simulink model "Testing_model"  (R2024b)
settings: Solver=FixedStepAuto  StartTime=0.0  StopTime=2  FixedStep=50e-6  RelTol=1e-3
undefined symbols (not defined in the file): alpha_Lpf, B, dspblkCoreblockFVToolHelper, gcbh, J, Ki_current, Ki_speed, Kp_current, Kp_speed, lamdaM, Ls, ma, P, Rs, T_max, Ts, Vdc
libraries: simulink x3, slpidlib x3, eeGeneralControl x1
settings Model: Creator=ahmed  LastModifiedBy=ahmed

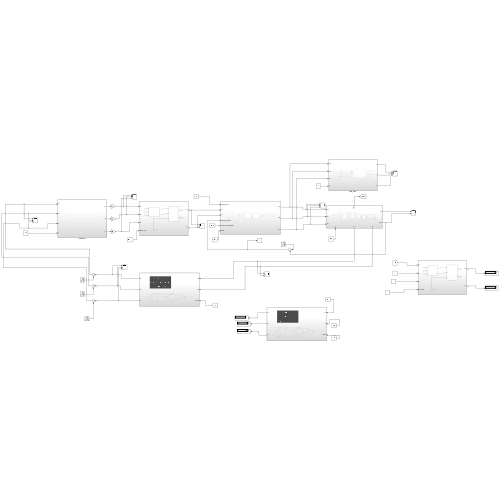
[thumbnail: Simulink's stored preview of the top-level diagram]
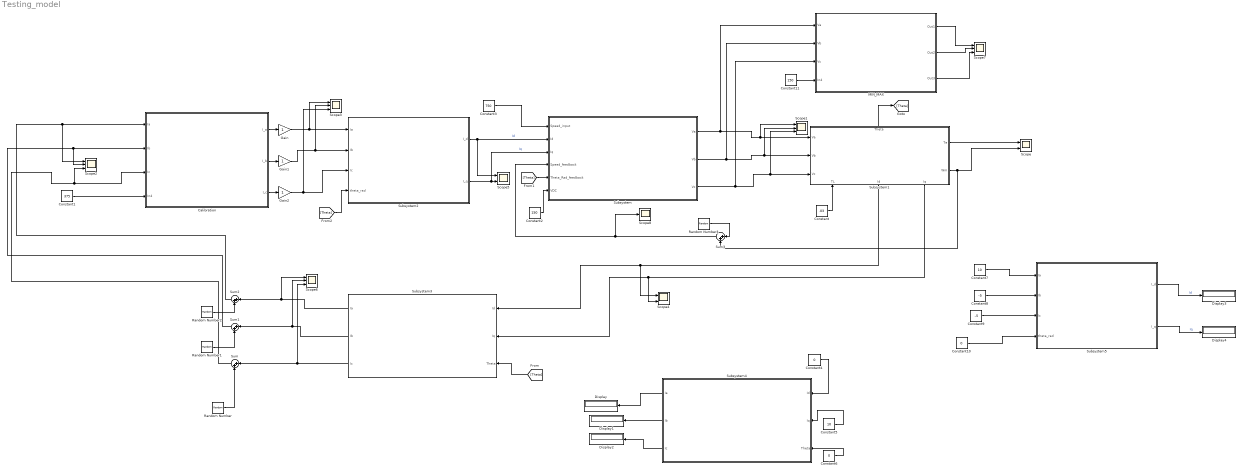
== system Testing_model ==
  Calibration : Subsystem
  Constant : Constant  Value=.03
  Constant1 : Constant  Value=375
  Constant10 : Constant  Value=0
  Constant11 : Constant  Value=150
  Constant2 : Constant  Value=150
  Constant3 : Constant  Value=750
  Constant4 : Constant  Value=0
  Constant5 : Constant  Value=10
  Constant6 : Constant  Value=0
  Constant7 : Constant  Value=10
  Constant8 : Constant  Value=-5
  Constant9 : Constant  Value=-5
  Display{,1..4} (5 alike) : Display
  Gain : Gain
  Gain1 : Gain
  Gain2 : Gain
  MIN_MAX : Subsystem
  Random Number : RandomNumber  Variance=.005  SampleTime=Ts
  Random Number1 : RandomNumber  Variance=.005  SampleTime=Ts
  Random Number2 : RandomNumber  Variance=.005  SampleTime=Ts
  Random Number3 : RandomNumber  Variance=50  SampleTime=Ts
  Scope : Scope  NumInputPorts=2
  Scope{1..3,6..7} (5 alike) : Scope  NumInputPorts=3
  Scope4 : Scope  NumInputPorts=2
  Scope5 : Scope  NumInputPorts=2
  Scope8 : Scope
  Subsystem : Subsystem
  Subsystem1 : Subsystem
      settings: PortSchema="{\"entries\":[{\"content\":{\"sides\":[{\"content\":{\"connectorIds\":[\"In1\",\"In2\",\"In3\"]},\"type\":\"ConnectorPlacement.EquallySpacedRectSide\",\"uuid\":\"410fafe1-6d3d-4b62-9ccb-454f6008b81a\"},{\"content\":{\"connectorIds\":[\"Out1\",\"Out2\"],\"side\":\"RIGHT\"},\"type\":\"ConnectorPlacement.EquallySpacedRectSide\",\"uuid\":\"b4215a85-6f2a-4bbd-a305-1fa3c25faaac\"},{\"content\":{\"connectorIds\":[\"Out5\"],\"side\":\"TOP\"},\"type\":\"ConnectorPlacement.EquallySpacedRectSide\",\"uuid\":\"c3471a58-e27d-4fa8-ab5e-4301d929309b\"},{\"content\":{\"connectorIds\":[\"In4\",\"Out3\",\"Out4\"],\"side\":\"BOTTOM\"},\"type\":\"ConnectorPlacement.EquallySpacedRectSide\",\"uuid\":\"92e7eecc-1ce6-457d-b998-008a2505e29d\"}]},\"type\":\"ConnectorPlacement.EquallySpacedConnector\",\"uuid\":\"8b1e994c-6614-4fb4-bf28-22b9fb88c59f\"}],\"packageUris\":[\"http://schema.mathworks.com/mf0/Connector/R2020b\"],\"version\":\"1.0\"}"
  Subsystem2 : Subsystem
  Subsystem3 : Subsystem
  Subsystem4 : Subsystem
  Subsystem5 : Subsystem
  Sum{,1..3} (4 alike) : Sum  Inputs=|++
  wires:
  Subsystem/1(Va) -> MIN_MAX/1(Va), Scope1/1, Subsystem1/1(Va)
  Subsystem/2(Vb) -> MIN_MAX/2(Vb), Scope1/2, Subsystem1/2(Vb)
  Subsystem/3(Vc) -> MIN_MAX/3(Vc), Scope1/3, Subsystem1/3(Vc)
  Subsystem1/5(Theta) -> [Theta]
  Constant/1 -> Subsystem1/4(TL)
  Subsystem1/1(Te) -> Scope/1
  Subsystem1/2(Wm) -> Scope/2, Sum3/2
  [Theta] -> Subsystem3/3(Theta)
  Constant1/1 -> Calibration/4(In4)
  [Theta] -> Subsystem/5(Theta_Rad_feedback)
  Constant2/1 -> Subsystem/6(VDC)
  Constant3/1 -> Subsystem/1(Speed_input)
  Random Number/1 -> Sum/2
  Subsystem3/3(Ic) -> Scope6/3, Sum/1
  Subsystem3/2(Ib) -> Sum1/1, Scope6/2
  Random Number1/1 -> Sum1/2
  Subsystem3/1(Ia) -> Scope6/1, Sum2/1
  Random Number2/1 -> Sum2/2
  [Theta] -> Subsystem2/4(theta_rad)
  Subsystem1/3(Id) -> Scope4/1, Subsystem3/1(Id)
  Subsystem1/4(Iq) -> Scope4/2, Subsystem3/2(Iq)
  Sum2/1 -> Scope2/1, Calibration/1(Ia)
  Sum1/1 -> Scope2/2, Calibration/2(Ib)
  Sum/1 -> Scope2/3, Calibration/3(Ic)
  Subsystem2/1(I_d) -> Scope5/1, Subsystem/2(Id)  "Id"
  Subsystem2/2(I_q) -> Scope5/2, Subsystem/3(Iq)  "Iq"
  Constant4/1 -> Subsystem4/1(Id)
  Constant5/1 -> Subsystem4/2(Iq)
  Constant6/1 -> Subsystem4/3(Theta)
  Subsystem4/1(Ia) -> Display/1
  Subsystem4/2(Ib) -> Display1/1
  Subsystem4/3(Ic) -> Display2/1
  Constant7/1 -> Subsystem5/1(Ia)
  Constant9/1 -> Subsystem5/3(Ic)
  Constant8/1 -> Subsystem5/2(Ib)
  Constant10/1 -> Subsystem5/4(theta_rad)
  Subsystem5/1(I_d) -> Display3/1  "Id"
  Subsystem5/2(I_q) -> Display4/1  "Iq"
  Calibration/2(I_b) -> Gain1/1
  Calibration/1(I_a) -> Gain/1
  Calibration/3(I_c) -> Gain2/1
  Gain/1 -> Subsystem2/1(Ia), Scope3/1
  Gain1/1 -> Scope3/2, Subsystem2/2(Ib)
  Gain2/1 -> Subsystem2/3(Ic), Scope3/3
  Constant11/1 -> MIN_MAX/4(In4)
  MIN_MAX/1(Out1) -> Scope7/1
  MIN_MAX/2(Out2) -> Scope7/2
  MIN_MAX/3(Out3) -> Scope7/3
  Sum3/1 -> Scope8/1, Subsystem/4(Speed_feedback)
  Random Number3/1 -> Sum3/1

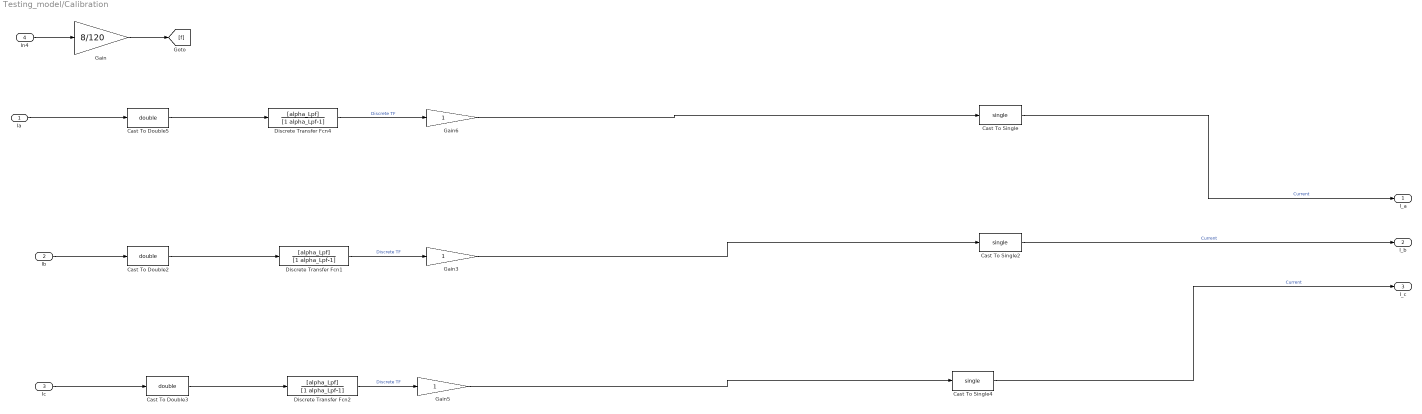
== system Testing_model/Calibration ==
  Ia : Inport
  Ib : Inport  Port=2
  Ic : Inport  Port=3
  In4 : Inport  Port=4
  Cast To Double2 : DataTypeConversion  OutDataTypeStr=double  SaturateOnIntegerOverflow=off  RndMeth=Floor
  Cast To Double3 : DataTypeConversion  OutDataTypeStr=double  SaturateOnIntegerOverflow=off  RndMeth=Floor
  Cast To Double5 : DataTypeConversion  OutDataTypeStr=double  SaturateOnIntegerOverflow=off  RndMeth=Floor
  Cast To Single : DataTypeConversion  OutDataTypeStr=single  SaturateOnIntegerOverflow=off  RndMeth=Floor
  Cast To Single2 : DataTypeConversion  OutDataTypeStr=single  SaturateOnIntegerOverflow=off  RndMeth=Floor
  Cast To Single4 : DataTypeConversion  OutDataTypeStr=single  SaturateOnIntegerOverflow=off  RndMeth=Floor
  Discrete Transfer Fcn1 : DiscreteTransferFcn  LoadFcn=dspblkCoreblockFVToolHelper(gcbh,'load');  Numerator=[alpha_Lpf]  Denominator=[1 alpha_Lpf-1]  RndMeth=Nearest
      settings: CopyFcn=dspblkCoreblockFVToolHelper(gcbh,'copy');  DeleteFcn=dspblkCoreblockFVToolHelper(gcbh,'close');  ModelCloseFcn=dspblkCoreblockFVToolHelper(gcbh,'close');  PreSaveFcn=dspblkCoreblockFVToolHelper(gcbh,'presave');  PostSaveFcn=dspblkCoreblockFVToolHelper(gcbh,'postsave');  CloseFcn=dspblkCoreblockFVToolHelper(gcbh,'close');
  Discrete Transfer Fcn2 : DiscreteTransferFcn  LoadFcn=dspblkCoreblockFVToolHelper(gcbh,'load');  Numerator=[alpha_Lpf]  Denominator=[1 alpha_Lpf-1]  RndMeth=Nearest
      settings: CopyFcn=dspblkCoreblockFVToolHelper(gcbh,'copy');  DeleteFcn=dspblkCoreblockFVToolHelper(gcbh,'close');  ModelCloseFcn=dspblkCoreblockFVToolHelper(gcbh,'close');  PreSaveFcn=dspblkCoreblockFVToolHelper(gcbh,'presave');  PostSaveFcn=dspblkCoreblockFVToolHelper(gcbh,'postsave');  CloseFcn=dspblkCoreblockFVToolHelper(gcbh,'close');
  Discrete Transfer Fcn4 : DiscreteTransferFcn  LoadFcn=dspblkCoreblockFVToolHelper(gcbh,'load');  Numerator=[alpha_Lpf]  Denominator=[1 alpha_Lpf-1]  RndMeth=Nearest
      settings: CopyFcn=dspblkCoreblockFVToolHelper(gcbh,'copy');  DeleteFcn=dspblkCoreblockFVToolHelper(gcbh,'close');  ModelCloseFcn=dspblkCoreblockFVToolHelper(gcbh,'close');  PreSaveFcn=dspblkCoreblockFVToolHelper(gcbh,'presave');  PostSaveFcn=dspblkCoreblockFVToolHelper(gcbh,'postsave');  CloseFcn=dspblkCoreblockFVToolHelper(gcbh,'close');
  Gain : Gain  Gain=8/120
  Gain3 : Gain
  Gain5 : Gain
  Gain6 : Gain
  I_a : Outport
  I_b : Outport  Port=2
  I_c : Outport  Port=3
  wires:
  Ib/1 -> Cast To Double2/1
  Gain3/1 -> Cast To Single2/1
  Discrete Transfer Fcn1/1 -> Gain3/1  "Discrete TF"
  Gain6/1 -> Cast To Single/1
  Gain5/1 -> Cast To Single4/1
  Cast To Double2/1 -> Discrete Transfer Fcn1/1
  Discrete Transfer Fcn4/1 -> Gain6/1  "Discrete TF"
  Cast To Double5/1 -> Discrete Transfer Fcn4/1
  Discrete Transfer Fcn2/1 -> Gain5/1  "Discrete TF"
  Cast To Single2/1 -> I_b/1  "Current"
  Cast To Double3/1 -> Discrete Transfer Fcn2/1
  Ia/1 -> Cast To Double5/1
  Cast To Single/1 -> I_a/1  "Current"
  Cast To Single4/1 -> I_c/1  "Current"
  Ic/1 -> Cast To Double3/1
  In4/1 -> Gain/1
  Gain/1 -> [f]

== system Testing_model/MIN_MAX ==
  Va : Inport
  Vb : Inport  Port=2
  Vc : Inport  Port=3
  In4 : Inport  Port=4
  Divide : Product  Inputs=*/
  Divide1 : Product  Inputs=*/
  Divide2 : Product  Inputs=*/
  Gain : Gain  Gain=1/sqrt(3)
  MIN_MAX : Subsystem
  Saturation : Saturate  UpperLimit=95  LowerLimit=0
  Saturation1 : Saturate  UpperLimit=95  LowerLimit=0
  Saturation2 : Saturate  UpperLimit=95  LowerLimit=0
  Scope2 : Scope  NumInputPorts=3
  Out1 : Outport
  Out2 : Outport  Port=2
  Out3 : Outport  Port=3
  wires:
  Saturation/1 -> Out1/1
  Saturation1/1 -> Out2/1
  Saturation2/1 -> Out3/1
  Va/1 -> Divide2/1
  Vb/1 -> Divide1/1
  Vc/1 -> Divide/1
  Divide2/1 -> MIN_MAX/1(In1), Scope2/1
  Divide1/1 -> Scope2/2, MIN_MAX/2(In2)
  Divide/1 -> Scope2/3, MIN_MAX/3(In3)
  In4/1 -> Gain/1
  Gain/1 -> Divide2/2, Divide1/2, Divide/2
  MIN_MAX/1(Out1) -> Saturation/1
  MIN_MAX/2(Out2) -> Saturation1/1
  MIN_MAX/3(Out3) -> Saturation2/1

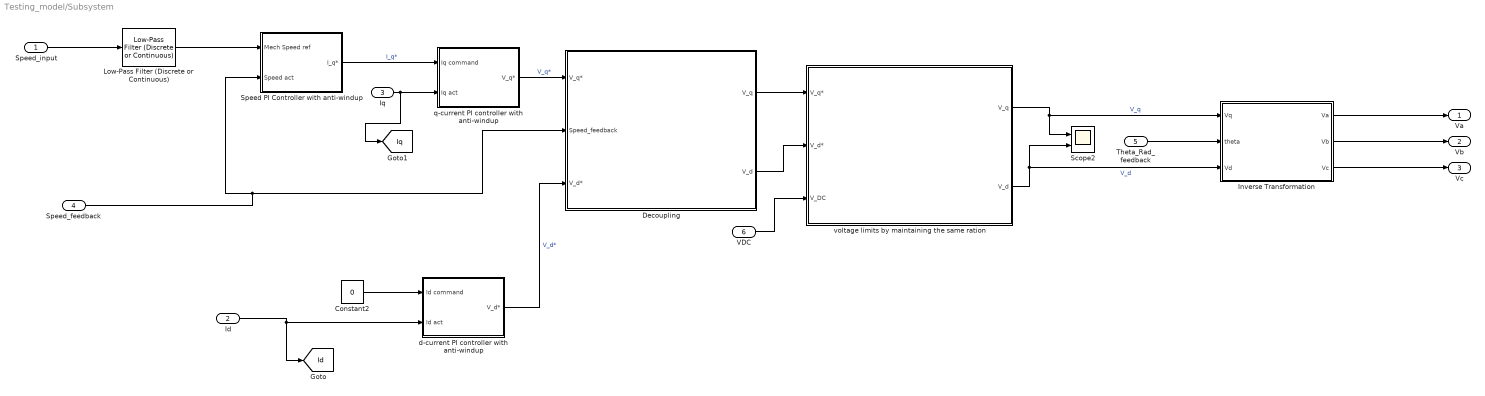
== system Testing_model/Subsystem ==
  Speed_input : Inport
  Id : Inport  Port=2
  Iq : Inport  Port=3
  Speed_feedback : Inport  Port=4
  Theta_Rad_feedback : Inport  Port=5
  VDC : Inport  Port=6
  Constant2 : Constant  Value=0  SampleTime=Ts
  Decoupling : Subsystem
  Inverse Transformation : Subsystem
  Low-Pass Filter (Discrete or Continuous) : eeGeneralControl/Low-Pass Filter (Discrete or Continuous)  K=1  T=1/60  B=inf  A=-inf  init_option=Inherited from block input  x0=0  Ts=-1
  Scope2 : Scope  NumInputPorts=2
  Speed PI Controller with anti-windup : Subsystem
  d-current PI controller with anti-windup : Subsystem
  q-current PI controller with anti-windup : Subsystem
  voltage limits by maintaining the same ration : Subsystem
  Va : Outport
  Vb : Outport  Port=2
  Vc : Outport  Port=3
  tag scope: Id=global, Iq=global
  wires:
  Speed_feedback/1 -> Decoupling/2(Speed_feedback), Speed PI Controller with anti-windup/2(Speed act)
  Speed_input/1 -> Low-Pass Filter (Discrete or Continuous)/1
  Iq/1 -> q-current PI controller with anti-windup/2(Iq act), [Iq]
  Speed PI Controller with anti-windup/1(I_q*) -> q-current PI controller with anti-windup/1(Iq command)  "I_q*"
  Constant2/1 -> d-current PI controller with anti-windup/1(Id command)
  Decoupling/2(V_d) -> voltage limits by maintaining the same ration/2(V_d*)
  Id/1 -> d-current PI controller with anti-windup/2(Id act), [Id]
  q-current PI controller with anti-windup/1(V_q*) -> Decoupling/1(V_q*)  "V_q*"
  d-current PI controller with anti-windup/1(V_d*) -> Decoupling/3(V_d*)  "V_d*"
  Decoupling/1(V_q) -> voltage limits by maintaining the same ration/1(V_q*)
  VDC/1 -> voltage limits by maintaining the same ration/3(V_DC)
  voltage limits by maintaining the same ration/1(V_q) -> Scope2/1, Inverse Transformation/1(Vq)  "V_q"
  voltage limits by maintaining the same ration/2(V_d) -> Inverse Transformation/3(Vd), Scope2/2  "V_d"
  Theta_Rad_feedback/1 -> Inverse Transformation/2(theta)
  Inverse Transformation/3(Vc) -> Vc/1
  Inverse Transformation/1(Va) -> Va/1
  Inverse Transformation/2(Vb) -> Vb/1
  Low-Pass Filter (Discrete or Continuous)/1 -> Speed PI Controller with anti-windup/1(Mech Speed ref)

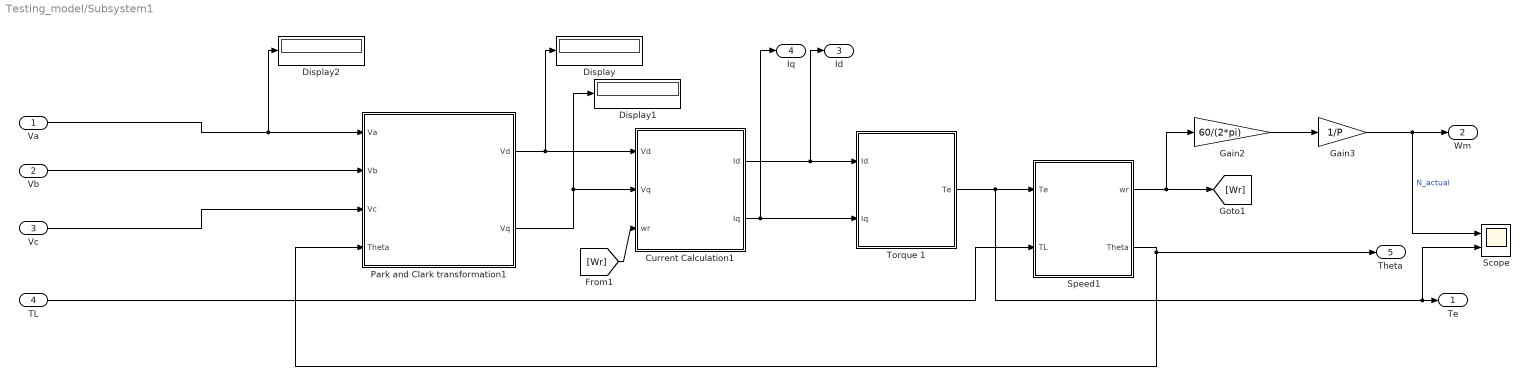
== system Testing_model/Subsystem1 ==
  Va : Inport
  Vb : Inport  Port=2
  Vc : Inport  Port=3
  TL : Inport  Port=4
  Current Calculation1 : Subsystem
  Display : Display
  Display1 : Display
  Display2 : Display
  Gain2 : Gain  Gain=60/(2*pi)
  Gain3 : Gain  Gain=1/P
  Park and Clark transformation1 : Subsystem
  Scope : Scope  NumInputPorts=2
  Speed1 : Subsystem
  Torque 1 : Subsystem
  Te : Outport
  Wm : Outport  Port=2
  Id : Outport  Port=3
  Iq : Outport  Port=4
  Theta : Outport  Port=5
  wires:
  [Wr] -> Current Calculation1/3(wr)
  Va/1 -> Display2/1, Park and Clark transformation1/1(Va)
  Park and Clark transformation1/2(Vq) -> Current Calculation1/2(Vq), Display1/1
  Torque 1/1(Te) -> Scope/2, Te/1, Speed1/1(Te)
  Speed1/1(wr) -> Gain2/1, [Wr]
  Park and Clark transformation1/1(Vd) -> Display/1, Current Calculation1/1(Vd)
  Gain2/1 -> Gain3/1
  Speed1/2(Theta) -> Park and Clark transformation1/4(Theta), Theta/1
  Current Calculation1/2(Iq) -> Torque 1/2(Iq), Iq/1
  Current Calculation1/1(Id) -> Id/1, Torque 1/1(Id)
  Vb/1 -> Park and Clark transformation1/2(Vb)
  Gain3/1 -> Scope/1, Wm/1  "N_actual"
  Vc/1 -> Park and Clark transformation1/3(Vc)
  TL/1 -> Speed1/2(TL)

== system Testing_model/Subsystem2 ==
  Ia : Inport
  Ib : Inport  Port=2
  Ic : Inport  Port=3
  theta_rad : Inport  Port=4
  Forward Clacke : Subsystem
  Forward Park : Subsystem
  I_d : Outport
  I_q : Outport  Port=2
  wires:
  Ic/1 -> Forward Clacke/3(Ic)
  Forward Clacke/2(I_beta) -> Forward Park/2(I_beta)
  Forward Clacke/1(I_alpha) -> Forward Park/1(I_alpha)
  Ia/1 -> Forward Clacke/1(Ia)
  Forward Park/1(I_d) -> I_d/1
  Forward Park/2(I_q) -> I_q/1
  Ib/1 -> Forward Clacke/2(Ib)
  theta_rad/1 -> Forward Park/3(theta_rad)

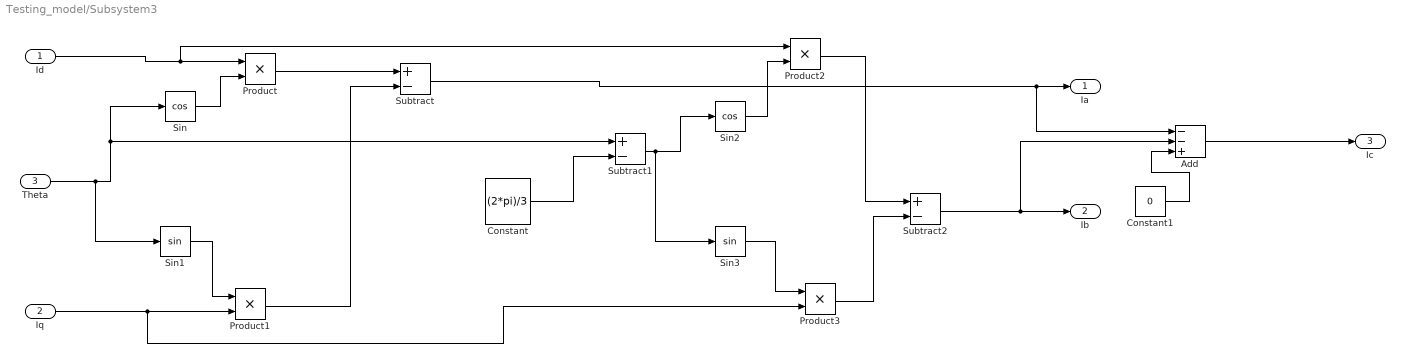
== system Testing_model/Subsystem3 ==
  Id : Inport
  Iq : Inport  Port=2
  Theta : Inport  Port=3
  Add : Sum  Inputs=--+
  Constant : Constant  Value=(2*pi)/3
  Constant1 : Constant  Value=0
  Product{,1..3} (4 alike) : Product
  Sin : Trigonometry  Operator=cos
  Sin1 : Trigonometry
  Sin2 : Trigonometry  Operator=cos
  Sin3 : Trigonometry
  Subtract : Sum  Inputs=+-
  Subtract1 : Sum  Inputs=+-
  Subtract2 : Sum  Inputs=+-
  Ia : Outport
  Ib : Outport  Port=2
  Ic : Outport  Port=3
  wires:
  Theta/1 -> Sin1/1, Sin/1, Subtract1/1
  Id/1 -> Product2/1, Product/1
  Sin/1 -> Product/2
  Product/1 -> Subtract/1
  Iq/1 -> Product3/2, Product1/2
  Sin1/1 -> Product1/1
  Product1/1 -> Subtract/2
  Subtract/1 -> Add/1, Ia/1
  Constant/1 -> Subtract1/2
  Subtract1/1 -> Sin3/1, Sin2/1
  Sin2/1 -> Product2/2
  Sin3/1 -> Product3/1
  Product3/1 -> Subtract2/2
  Product2/1 -> Subtract2/1
  Subtract2/1 -> Add/2, Ib/1
  Constant1/1 -> Add/3
  Add/1 -> Ic/1

== system Testing_model/Subsystem4 ==
  Id : Inport
  Iq : Inport  Port=2
  Theta : Inport  Port=3
  Add : Sum  Inputs=--+
  Constant : Constant  Value=(2*pi)/3
  Constant1 : Constant  Value=0
  Product{,1..3} (4 alike) : Product
  Sin : Trigonometry  Operator=cos
  Sin1 : Trigonometry
  Sin2 : Trigonometry  Operator=cos
  Sin3 : Trigonometry
  Subtract : Sum  Inputs=+-
  Subtract1 : Sum  Inputs=+-
  Subtract2 : Sum  Inputs=+-
  Ia : Outport
  Ib : Outport  Port=2
  Ic : Outport  Port=3
  wires:
  Add/1 -> Ic/1
  Constant1/1 -> Add/3
  Subtract2/1 -> Ib/1, Add/2
  Product2/1 -> Subtract2/1
  Product3/1 -> Subtract2/2
  Sin3/1 -> Product3/1
  Sin2/1 -> Product2/2
  Subtract1/1 -> Sin2/1, Sin3/1
  Constant/1 -> Subtract1/2
  Subtract/1 -> Ia/1, Add/1
  Product1/1 -> Subtract/2
  Sin1/1 -> Product1/1
  Iq/1 -> Product1/2, Product3/2
  Product/1 -> Subtract/1
  Sin/1 -> Product/2
  Id/1 -> Product/1, Product2/1
  Theta/1 -> Subtract1/1, Sin/1, Sin1/1

== system Testing_model/Subsystem5 ==
  Ia : Inport
  Ib : Inport  Port=2
  Ic : Inport  Port=3
  theta_rad : Inport  Port=4
  Forward Clacke : Subsystem
  Forward Park : Subsystem
  I_d : Outport
  I_q : Outport  Port=2
  wires:
  theta_rad/1 -> Forward Park/3(theta_rad)
  Ib/1 -> Forward Clacke/2(Ib)
  Forward Park/2(I_q) -> I_q/1
  Forward Park/1(I_d) -> I_d/1
  Ia/1 -> Forward Clacke/1(Ia)
  Forward Clacke/1(I_alpha) -> Forward Park/1(I_alpha)
  Forward Clacke/2(I_beta) -> Forward Park/2(I_beta)
  Ic/1 -> Forward Clacke/3(Ic)

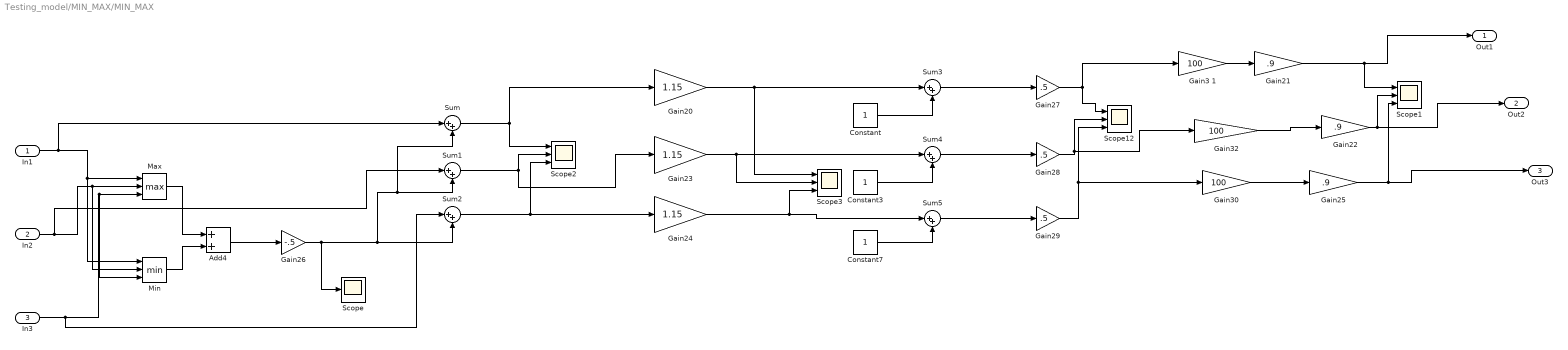
== system Testing_model/MIN_MAX/MIN_MAX ==
  In1 : Inport
  In2 : Inport  Port=2
  In3 : Inport  Port=3
  Add4 : Sum
  Constant : Constant
  Constant3 : Constant
  Constant7 : Constant
  Gain20 : Gain  Gain=1.15
  Gain21 : Gain  Gain=.9
  Gain22 : Gain  Gain=.9
  Gain23 : Gain  Gain=1.15
  Gain24 : Gain  Gain=1.15
  Gain25 : Gain  Gain=.9
  Gain26 : Gain  Gain=-.5
  Gain27 : Gain  Gain=.5
  Gain28 : Gain  Gain=.5
  Gain29 : Gain  Gain=.5
  Gain3 1 : Gain  Gain=100
  Gain30 : Gain  Gain=100
  Gain32 : Gain  Gain=100
  Max : MinMax  Function=max  Inputs=3
  Min : MinMax  Inputs=3
  Scope : Scope
  Scope{1..3,12} (4 alike) : Scope  NumInputPorts=3
  Sum{,1..5} (6 alike) : Sum  Inputs=|++
  Out1 : Outport
  Out2 : Outport  Port=2
  Out3 : Outport  Port=3
  wires:
  Gain28/1 -> Scope12/2, Gain32/1
  Sum3/1 -> Gain27/1
  In1/1 -> Sum/1, Min/1, Max/1
  Gain32/1 -> Gain22/1
  In3/1 -> Sum2/1, Min/3, Max/3
  Gain29/1 -> Scope12/3, Gain30/1
  In2/1 -> Sum1/1, Min/2, Max/2
  Constant7/1 -> Sum5/2
  Gain26/1 -> Scope/1, Sum/2, Sum1/2, Sum2/2
  Add4/1 -> Gain26/1
  Gain30/1 -> Gain25/1
  Min/1 -> Add4/2
  Gain20/1 -> Scope3/1, Sum3/1
  Gain27/1 -> Scope12/1, Gain3 1/1
  Constant3/1 -> Sum4/2
  Gain24/1 -> Scope3/3, Sum5/1
  Constant/1 -> Sum3/2
  Sum4/1 -> Gain28/1
  Sum1/1 -> Scope2/2, Gain23/1
  Max/1 -> Add4/1
  Gain25/1 -> Scope1/3, Out3/1
  Gain3 1/1 -> Gain21/1
  Sum2/1 -> Scope2/3, Gain24/1
  Gain23/1 -> Scope3/2, Sum4/1
  Sum5/1 -> Gain29/1
  Gain22/1 -> Scope1/2, Out2/1
  Gain21/1 -> Scope1/1, Out1/1
  Sum/1 -> Scope2/1, Gain20/1

== system Testing_model/Subsystem/Decoupling ==
  V_q* : Inport
  Speed_feedback : Inport  Port=2
  V_d* : Inport  Port=3
  Gain : Gain  Gain=(2*pi)/60
  Gain1 : Gain  Gain=P
  Gain2 : Gain  Gain=P
  Gain3 : Gain  Gain=P
  Lambda_m : Constant  Value=lamdaM
  Lambda_m1 : Constant  Value=lamdaM
  Ld : Constant  Value=Ls
  Product : Product  Inputs=3
  Product1 : Product
  Product2 : Product  Inputs=3
  Sum3 : Sum  Inputs=+++
  Sum4 : Sum  Inputs=|+-
  V_q : Outport
  V_d : Outport  Port=2
  wires:
  [Iq] -> Product2/1
  [Id] -> Product/1
  Product2/1 -> Sum4/2
  Gain3/1 -> Product1/1
  Gain2/1 -> Product/2
  Product1/1 -> Sum3/3
  Gain1/1 -> Product2/2
  Gain/1 -> Gain3/1, Gain1/1, Gain2/1
  Lambda_m/1 -> Product1/2
  Ld/1 -> Product/3
  Sum4/1 -> V_d/1
  Lambda_m1/1 -> Product2/3
  Product/1 -> Sum3/1
  V_q*/1 -> Sum3/2
  Sum3/1 -> V_q/1
  V_d*/1 -> Sum4/1
  Speed_feedback/1 -> Gain/1

== system Testing_model/Subsystem/Inverse Transformation ==
  Vq : Inport
  theta : Inport  Port=2
  Vd : Inport  Port=3
  Cast To Single : DataTypeConversion  OutDataTypeStr=single  SaturateOnIntegerOverflow=off  RndMeth=Floor
  Cast To Single1 : DataTypeConversion  OutDataTypeStr=single  SaturateOnIntegerOverflow=off  RndMeth=Floor
  Cast To Single2 : DataTypeConversion  OutDataTypeStr=single  SaturateOnIntegerOverflow=off  RndMeth=Floor
  "Inverse Park " : Subsystem  Commented=on
  dq to abc : Subsystem
  inverse Clark : Subsystem  Commented=on
  Va : Outport
  Vb : Outport  Port=2
  Vc : Outport  Port=3
  wires:
  theta/1 -> dq to abc/3(theta)
  Vq/1 -> dq to abc/1(V_q*)
  Vd/1 -> dq to abc/2(V_d*)
  dq to abc/1(Va*) -> Cast To Single/1
  dq to abc/2(Vb*) -> Cast To Single1/1
  dq to abc/3(Vc*) -> Cast To Single2/1
  Cast To Single/1 -> Va/1
  Cast To Single1/1 -> Vb/1
  Cast To Single2/1 -> Vc/1

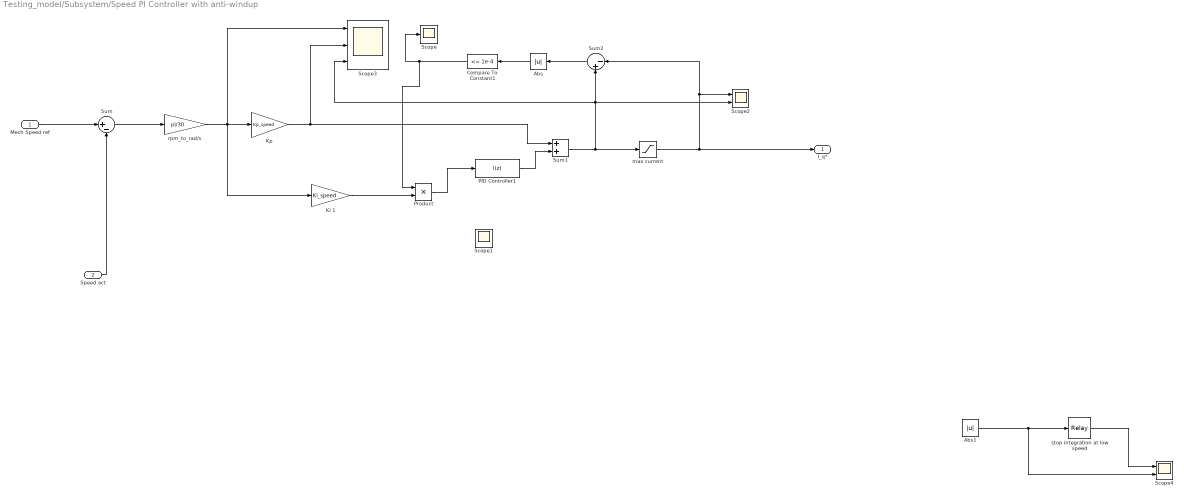
== system Testing_model/Subsystem/Speed PI Controller with anti-windup ==
  Mech Speed ref : Inport
  Speed act : Inport  Port=2
  " max current" : Saturate  UpperLimit=T_max/((3/2)*lamdaM*P)  LowerLimit=-T_max/((3/2)*lamdaM*P)
  Abs : Abs  SaturateOnIntegerOverflow=off
  Abs1 : Abs  SaturateOnIntegerOverflow=off
  Compare To Constant1 : simulink/Logic and Bit Operations/Compare To Constant  relop=<=  const=1e-4  OutDataTypeStr=boolean
  Ki 1 : Gain  Gain=Ki_speed
  Kp : Gain  Gain=Kp_speed
  PID Controller1 : slpidlib/PID Controller  Controller=I  Form=Parallel  TimeDomain=Discrete-time  UseExternalTs=off  SampleTime=Ts  IntegratorMethod=Forward Euler  FilterMethod=Forward Euler  ControllerParametersSource=internal  P=1  I=1  UseKiTs=off  D=0  UseExternalDerivativeSource=off  N=100  UseFilter=on  TunerSelectOption=Transfer Function Based (PID Tuner App)  InitialConditionSource=internal  InitialConditionForIntegrator=0  InitialConditionForFilter=0  DifferentiatorICPrevScaledInput=0  ExternalReset=none  TrackingMode=off  Kt=1  LimitOutput=on  SatLimitsSource=internal  UpperSaturationLimit=T_max/((3/2)*lamdaM*P)  LowerSaturationLimit=-T_max/((3/2)*lamdaM*P)  LinearizeAsGain=on  AntiWindupMode=clamping  Kb=1  LimitIntegrator=off  UpperIntegratorSaturationLimit=inf  LowerIntegratorSaturationLimit=-inf  POutMin=[]  POutMax=[]  IOutMin=[]  IOutMax=[]  DOutMin=[]  DOutMax=[]  NOutMin=[]  NOutMax=[]  SumOutMin=[]  SumOutMax=[]  SaturationOutMin=[]  SaturationOutMax=[]  PParamMin=[]  PParamMax=[]  IParamMin=[]  IParamMax=[]  DParamMin=[]  DParamMax=[]  NParamMin=[]  NParamMax=[]  KbParamMin=[]  KbParamMax=[]  KtParamMin=[]  KtParamMax=[]  KbOutMin=[]  KbOutMax=[]  KtOutMin=[]  KtOutMax=[]  IntegratorOutMin=[]  IntegratorOutMax=[]  FilterOutMin=[]  FilterOutMax=[]  SumI1OutMin=[]  SumI1OutMax=[]  SumI2OutMin=[]  SumI2OutMax=[]  SumI3OutMin=[]  SumI3OutMax=[]  SumI4OutMin=[]  SumI4OutMax=[]  SumDOutMin=[]  SumDOutMax=[]  DifferentiatorOutMin=[]  DifferentiatorOutMax=[]  FilterDiffOutCoefMin=[]  FilterDiffOutCoefMax=[]  ReciprocalOutMin=[]  ReciprocalOutMax=[]  SumDenOutMin=[]  SumDenOutMax=[]  SumNumOutMin=[]  SumNumOutMax=[]  DivideOutMin=[]  DivideOutMax=[]  UdiffTsProdOutMin=[]  UdiffTsProdOutMax=[]  NTsProdOutMin=[]  NTsProdOutMax=[]  UintegralTsProdOutMin=[]  UintegralTsProdOutMax=[]  UngainTsProdOutMin=[]  UngainTsProdOutMax=[]  ClampingZeroOutDataTypeStr=Inherit: Inherit via back propagation  ClampingZeroOutMin=[]  ClampingZeroOutMax=[]  FilterDenConstantOutDataTypeStr=Inherit: Inherit via back propagation  FilterDenConstantOutMin=[]  FilterDenConstantOutMax=[]  PCopyOutDataTypeStr=Inherit: Inherit via back propagation  PCopyOutMin=[]  PCopyOutMax=[]  NCopyOutDataTypeStr=Inherit: Inherit via back propagation  NCopyOutMin=[]  NCopyOutMax=[]  IntegratorContinuousStateAttributes=''  IntegratorStateMustResolveToSignalObject=off  IntegratorRTWStateStorageClass=Auto  FilterContinuousStateAttributes=''  FilterStateMustResolveToSignalObject=off  FilterRTWStateStorageClass=Auto  ParallelPVariant=Disabled  IdealPVariant=Disabled  IVariant=InternalParameters  DVariant=Disabled  IntegratorVariant=Discrete  SatVariant=Enabled  AWVariant=DiscClampingParallel  PCopyVariant=Disabled  TRVariant=Disabled  FdbkBlocksVariant=Forward  IdealPFdbkVariant=Disabled  SatFdbkVariant=Disabled  DerivativeFilterVariant=Disabled  NVariant=Disabled  NCopyVariant=Disabled_SignalSpec  FilterICVariant=Disabled  IntegratorICVariant=InternalICs  ExternalResetVariant=Disabled  TRSumVariant=Passthrough  SumFdbkVariant=Disabled  SumVariant=Passthrough_I  TsampFilterVariant=InternalTs  TsampNgainVariant=Passthrough  TsampIntegralVariant=Disabled_SignalSpec  ExternalSaturationOutDataTypeStr=Inherit: Same as second input  DerivativeSourceVariant=Disabled  PreIntVariant=InternalPreInt
  Product : Product
  Scope : Scope
  Scope1 : Scope  NumInputPorts=2
  Scope2 : Scope  NumInputPorts=2
  Scope3 : Scope  NumInputPorts=3
  Scope4 : Scope  NumInputPorts=2
  Sum : Sum  Inputs=|+-
  Sum1 : Sum
  Sum2 : Sum  Inputs=|-+
  rpm_to_rad/s : Gain  Gain=pi/30
  stop integration at low speed : Relay  OnSwitchValue=100  OffSwitchValue=-100
  I_q* : Outport
  wires:
  " max current"/1 -> Scope2/1, Sum2/1, I_q*/1
  Sum/1 -> rpm_to_rad/s/1
  rpm_to_rad/s/1 -> Ki 1/1, Kp/1, Scope3/1
  stop integration at low speed/1 -> Scope4/1
  Abs1/1 -> Scope4/2, stop integration at low speed/1
  Compare To Constant1/1 -> Product/1, Scope/1
  Abs/1 -> Compare To Constant1/1
  Sum2/1 -> Abs/1
  Sum1/1 -> " max current"/1, Sum2/2, Scope3/3, Scope2/2
  Kp/1 -> Sum1/1, Scope3/2
  Speed act/1 -> Sum/2
  Mech Speed ref/1 -> Sum/1
  PID Controller1/1 -> Sum1/2
  Ki 1/1 -> Product/2
  Product/1 -> PID Controller1/1

== system Testing_model/Subsystem/d-current PI controller with anti-windup ==
  Id command : Inport
  Id act : Inport  Port=2
  I_controller : slpidlib/PID Controller  Controller=I  Form=Parallel  TimeDomain=Discrete-time  UseExternalTs=off  SampleTime=Ts  IntegratorMethod=Forward Euler  FilterMethod=Forward Euler  ControllerParametersSource=internal  P=1  I=1  UseKiTs=off  D=0  UseExternalDerivativeSource=off  N=100  UseFilter=on  TunerSelectOption=Transfer Function Based (PID Tuner App)  InitialConditionSource=internal  InitialConditionForIntegrator=0  InitialConditionForFilter=0  DifferentiatorICPrevScaledInput=0  ExternalReset=none  TrackingMode=off  Kt=1  LimitOutput=on  SatLimitsSource=internal  UpperSaturationLimit=Vdc/sqrt(3)  LowerSaturationLimit=-Vdc/sqrt(3)  LinearizeAsGain=on  AntiWindupMode=clamping  Kb=1  LimitIntegrator=off  UpperIntegratorSaturationLimit=inf  LowerIntegratorSaturationLimit=-inf  POutMin=[]  POutMax=[]  IOutMin=[]  IOutMax=[]  DOutMin=[]  DOutMax=[]  NOutMin=[]  NOutMax=[]  SumOutMin=[]  SumOutMax=[]  SaturationOutMin=[]  SaturationOutMax=[]  PParamMin=[]  PParamMax=[]  IParamMin=[]  IParamMax=[]  DParamMin=[]  DParamMax=[]  NParamMin=[]  NParamMax=[]  KbParamMin=[]  KbParamMax=[]  KtParamMin=[]  KtParamMax=[]  KbOutMin=[]  KbOutMax=[]  KtOutMin=[]  KtOutMax=[]  IntegratorOutMin=[]  IntegratorOutMax=[]  FilterOutMin=[]  FilterOutMax=[]  SumI1OutMin=[]  SumI1OutMax=[]  SumI2OutMin=[]  SumI2OutMax=[]  SumI3OutMin=[]  SumI3OutMax=[]  SumI4OutMin=[]  SumI4OutMax=[]  SumDOutMin=[]  SumDOutMax=[]  DifferentiatorOutMin=[]  DifferentiatorOutMax=[]  FilterDiffOutCoefMin=[]  FilterDiffOutCoefMax=[]  ReciprocalOutMin=[]  ReciprocalOutMax=[]  SumDenOutMin=[]  SumDenOutMax=[]  SumNumOutMin=[]  SumNumOutMax=[]  DivideOutMin=[]  DivideOutMax=[]  UdiffTsProdOutMin=[]  UdiffTsProdOutMax=[]  NTsProdOutMin=[]  NTsProdOutMax=[]  UintegralTsProdOutMin=[]  UintegralTsProdOutMax=[]  UngainTsProdOutMin=[]  UngainTsProdOutMax=[]  ClampingZeroOutDataTypeStr=Inherit: Inherit via back propagation  ClampingZeroOutMin=[]  ClampingZeroOutMax=[]  FilterDenConstantOutDataTypeStr=Inherit: Inherit via back propagation  FilterDenConstantOutMin=[]  FilterDenConstantOutMax=[]  PCopyOutDataTypeStr=Inherit: Inherit via back propagation  PCopyOutMin=[]  PCopyOutMax=[]  NCopyOutDataTypeStr=Inherit: Inherit via back propagation  NCopyOutMin=[]  NCopyOutMax=[]  IntegratorContinuousStateAttributes=''  IntegratorStateMustResolveToSignalObject=off  IntegratorRTWStateStorageClass=Auto  FilterContinuousStateAttributes=''  FilterStateMustResolveToSignalObject=off  FilterRTWStateStorageClass=Auto  ParallelPVariant=Disabled  IdealPVariant=Disabled  IVariant=InternalParameters  DVariant=Disabled  IntegratorVariant=Discrete  SatVariant=Enabled  AWVariant=DiscClampingParallel  PCopyVariant=Disabled  TRVariant=Disabled  FdbkBlocksVariant=Forward  IdealPFdbkVariant=Disabled  SatFdbkVariant=Disabled  DerivativeFilterVariant=Disabled  NVariant=Disabled  NCopyVariant=Disabled_SignalSpec  FilterICVariant=Disabled  IntegratorICVariant=InternalICs  ExternalResetVariant=Disabled  TRSumVariant=Passthrough  SumFdbkVariant=Disabled  SumVariant=Passthrough_I  TsampFilterVariant=InternalTs  TsampNgainVariant=Passthrough  TsampIntegralVariant=Disabled_SignalSpec  ExternalSaturationOutDataTypeStr=Inherit: Same as second input  DerivativeSourceVariant=Disabled  PreIntVariant=InternalPreInt
  Ki 1 : Gain  Gain=Ki_current
  Kp : Gain  Gain=Kp_current
  Product : Product
  Scope : Scope
  Scope2 : Scope  NumInputPorts=2
  Scope3 : Scope  NumInputPorts=3
  Sum : Sum  Inputs=|+-
  Sum1 : Sum
  V_d* : Outport
  wires:
  Sum1/1 -> V_d*/1, Scope3/3, Scope2/2
  Sum/1 -> Ki 1/1, Kp/1, Scope3/1
  Kp/1 -> Sum1/1, Scope3/2
  Id act/1 -> Sum/2
  Id command/1 -> Sum/1
  [stop_d_integrator] -> Product/1, Scope/1
  Ki 1/1 -> Product/2
  Product/1 -> I_controller/1
  I_controller/1 -> Sum1/2

== system Testing_model/Subsystem/q-current PI controller with anti-windup ==
  Iq command : Inport
  Iq act : Inport  Port=2
  I_controller : slpidlib/PID Controller  Controller=I  Form=Parallel  TimeDomain=Discrete-time  UseExternalTs=off  SampleTime=Ts  IntegratorMethod=Forward Euler  FilterMethod=Forward Euler  ControllerParametersSource=internal  P=1  I=1  UseKiTs=off  D=0  UseExternalDerivativeSource=off  N=100  UseFilter=on  TunerSelectOption=Transfer Function Based (PID Tuner App)  InitialConditionSource=internal  InitialConditionForIntegrator=0  InitialConditionForFilter=0  DifferentiatorICPrevScaledInput=0  ExternalReset=none  TrackingMode=off  Kt=1  LimitOutput=on  SatLimitsSource=internal  UpperSaturationLimit=Vdc/sqrt(3)  LowerSaturationLimit=-Vdc/sqrt(3)  LinearizeAsGain=on  AntiWindupMode=clamping  Kb=1  LimitIntegrator=off  UpperIntegratorSaturationLimit=inf  LowerIntegratorSaturationLimit=-inf  POutMin=[]  POutMax=[]  IOutMin=[]  IOutMax=[]  DOutMin=[]  DOutMax=[]  NOutMin=[]  NOutMax=[]  SumOutMin=[]  SumOutMax=[]  SaturationOutMin=[]  SaturationOutMax=[]  PParamMin=[]  PParamMax=[]  IParamMin=[]  IParamMax=[]  DParamMin=[]  DParamMax=[]  NParamMin=[]  NParamMax=[]  KbParamMin=[]  KbParamMax=[]  KtParamMin=[]  KtParamMax=[]  KbOutMin=[]  KbOutMax=[]  KtOutMin=[]  KtOutMax=[]  IntegratorOutMin=[]  IntegratorOutMax=[]  FilterOutMin=[]  FilterOutMax=[]  SumI1OutMin=[]  SumI1OutMax=[]  SumI2OutMin=[]  SumI2OutMax=[]  SumI3OutMin=[]  SumI3OutMax=[]  SumI4OutMin=[]  SumI4OutMax=[]  SumDOutMin=[]  SumDOutMax=[]  DifferentiatorOutMin=[]  DifferentiatorOutMax=[]  FilterDiffOutCoefMin=[]  FilterDiffOutCoefMax=[]  ReciprocalOutMin=[]  ReciprocalOutMax=[]  SumDenOutMin=[]  SumDenOutMax=[]  SumNumOutMin=[]  SumNumOutMax=[]  DivideOutMin=[]  DivideOutMax=[]  UdiffTsProdOutMin=[]  UdiffTsProdOutMax=[]  NTsProdOutMin=[]  NTsProdOutMax=[]  UintegralTsProdOutMin=[]  UintegralTsProdOutMax=[]  UngainTsProdOutMin=[]  UngainTsProdOutMax=[]  ClampingZeroOutDataTypeStr=Inherit: Inherit via back propagation  ClampingZeroOutMin=[]  ClampingZeroOutMax=[]  FilterDenConstantOutDataTypeStr=Inherit: Inherit via back propagation  FilterDenConstantOutMin=[]  FilterDenConstantOutMax=[]  PCopyOutDataTypeStr=Inherit: Inherit via back propagation  PCopyOutMin=[]  PCopyOutMax=[]  NCopyOutDataTypeStr=Inherit: Inherit via back propagation  NCopyOutMin=[]  NCopyOutMax=[]  IntegratorContinuousStateAttributes=''  IntegratorStateMustResolveToSignalObject=off  IntegratorRTWStateStorageClass=Auto  FilterContinuousStateAttributes=''  FilterStateMustResolveToSignalObject=off  FilterRTWStateStorageClass=Auto  ParallelPVariant=Disabled  IdealPVariant=Disabled  IVariant=InternalParameters  DVariant=Disabled  IntegratorVariant=Discrete  SatVariant=Enabled  AWVariant=DiscClampingParallel  PCopyVariant=Disabled  TRVariant=Disabled  FdbkBlocksVariant=Forward  IdealPFdbkVariant=Disabled  SatFdbkVariant=Disabled  DerivativeFilterVariant=Disabled  NVariant=Disabled  NCopyVariant=Disabled_SignalSpec  FilterICVariant=Disabled  IntegratorICVariant=InternalICs  ExternalResetVariant=Disabled  TRSumVariant=Passthrough  SumFdbkVariant=Disabled  SumVariant=Passthrough_I  TsampFilterVariant=InternalTs  TsampNgainVariant=Passthrough  TsampIntegralVariant=Disabled_SignalSpec  ExternalSaturationOutDataTypeStr=Inherit: Same as second input  DerivativeSourceVariant=Disabled  PreIntVariant=InternalPreInt
  Ki 1 : Gain  Gain=Ki_current
  Kp : Gain  Gain=Kp_current
  Product : Product
  Scope : Scope
  Scope2 : Scope  NumInputPorts=2
  Scope3 : Scope  NumInputPorts=3
  Sum : Sum  Inputs=|+-
  Sum1 : Sum
  V_q* : Outport
  wires:
  Iq command/1 -> Sum/1
  Iq act/1 -> Sum/2
  Sum/1 -> Ki 1/1, Scope3/1, Kp/1
  Kp/1 -> Scope3/2, Sum1/1
  Sum1/1 -> V_q*/1, Scope2/2, Scope3/3
  [stop_q_integrator] -> Product/1, Scope/1
  Ki 1/1 -> Product/2
  Product/1 -> I_controller/1
  I_controller/1 -> Sum1/2

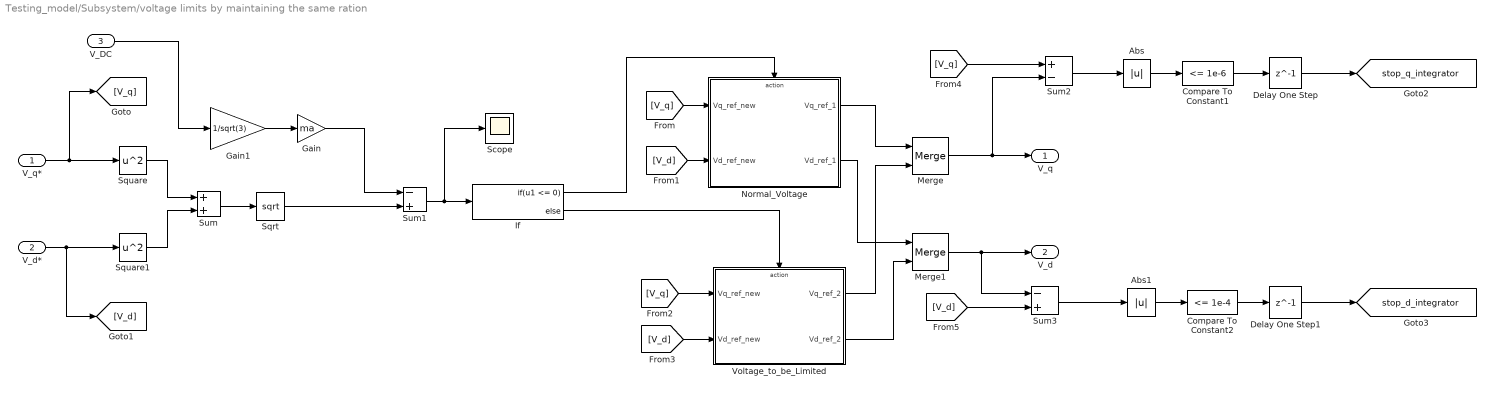
== system Testing_model/Subsystem/voltage limits by maintaining the same ration ==
  V_q* : Inport
  V_d* : Inport  Port=2
  V_DC : Inport  Port=3
  Abs : Abs  SaturateOnIntegerOverflow=off
  Abs1 : Abs  SaturateOnIntegerOverflow=off
  Compare To Constant1 : simulink/Logic and Bit Operations/Compare To Constant  relop=<=  const=1e-6  OutDataTypeStr=boolean
  Compare To Constant2 : simulink/Logic and Bit Operations/Compare To Constant  relop=<=  const=1e-4  OutDataTypeStr=boolean
  Delay One Step : Delay  DelayLength=1
  Delay One Step1 : Delay  DelayLength=1
  Gain : Gain  Gain=ma
  Gain1 : Gain  Gain=1/sqrt(3)
  If : If  IfExpression=u1 <= 0
  Merge : Merge
  Merge1 : Merge
  Normal_Voltage : Subsystem  TreatAsAtomicUnit=on
      settings: RTWSystemCode=Inline  RTWFcnNameOpts=Use subsystem name  RTWFileNameOpts=Use subsystem name
  Scope : Scope
  Sqrt : Sqrt
  Square : Math  Operator=square
  Square1 : Math  Operator=square
  Sum : Sum
  Sum1 : Sum  Inputs=-+
  Sum2 : Sum  Inputs=+-
  Sum3 : Sum  Inputs=-+
  Voltage_to_be_Limited : Subsystem  TreatAsAtomicUnit=on
      settings: RTWSystemCode=Inline  RTWFcnNameOpts=Use subsystem name  RTWFileNameOpts=Use subsystem name
  V_q : Outport
  V_d : Outport  Port=2
  tag scope: stop_d_integrator=global, stop_q_integrator=global
  wires:
  V_q*/1 -> [V_q], Square/1
  V_d*/1 -> [V_d], Square1/1
  Sum/1 -> Sqrt/1
  Square/1 -> Sum/1
  Square1/1 -> Sum/2
  Sqrt/1 -> Sum1/2
  Merge/1 -> Sum2/2, V_q/1
  Gain1/1 -> Gain/1
  Gain/1 -> Sum1/1
  Sum1/1 -> Scope/1, If/1
  If/1 -> Normal_Voltage/Action
  [V_q] -> Normal_Voltage/1(Vq_ref_new)
  [V_d] -> Normal_Voltage/2(Vd_ref_new)
  If/2 -> Voltage_to_be_Limited/Action
  Voltage_to_be_Limited/1(Vq_ref_2) -> Merge/2
  Normal_Voltage/1(Vq_ref_1) -> Merge/1
  Voltage_to_be_Limited/2(Vd_ref_2) -> Merge1/2
  Normal_Voltage/2(Vd_ref_1) -> Merge1/1
  [V_q] -> Voltage_to_be_Limited/1(Vq_ref_new)
  [V_d] -> Voltage_to_be_Limited/2(Vd_ref_new)
  [V_q] -> Sum2/1
  Merge1/1 -> Sum3/1, V_d/1
  [V_d] -> Sum3/2
  Delay One Step/1 -> [stop_q_integrator]
  Delay One Step1/1 -> [stop_d_integrator]
  Abs/1 -> Compare To Constant1/1
  Compare To Constant1/1 -> Delay One Step/1
  Sum2/1 -> Abs/1
  Sum3/1 -> Abs1/1
  Abs1/1 -> Compare To Constant2/1
  Compare To Constant2/1 -> Delay One Step1/1
  V_DC/1 -> Gain1/1

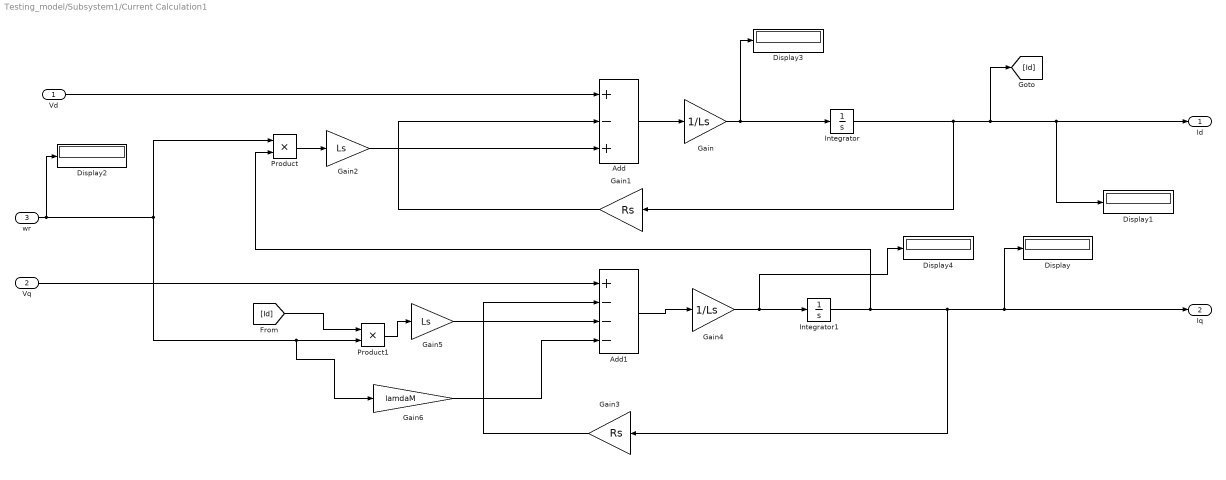
== system Testing_model/Subsystem1/Current Calculation1 ==
  Vd : Inport
  Vq : Inport  Port=2
  wr : Inport  Port=3
  Add : Sum  Inputs=+-+
  Add1 : Sum  Inputs=+---
  Display{,1..4} (5 alike) : Display
  Gain : Gain  Gain=1/Ls
  Gain1 : Gain  Gain=Rs
  Gain2 : Gain  Gain=Ls
  Gain3 : Gain  Gain=Rs
  Gain4 : Gain  Gain=1/Ls
  Gain5 : Gain  Gain=Ls
  Gain6 : Gain  Gain=lamdaM
  Integrator : Integrator
  Integrator1 : Integrator
  Product : Product
  Product1 : Product
  Id : Outport
  Iq : Outport  Port=2
  wires:
  Gain6/1 -> Add1/4
  Gain5/1 -> Add1/3
  Product1/1 -> Gain5/1
  [Id] -> Product1/1
  Gain3/1 -> Add1/2
  Integrator1/1 -> Gain3/1, Iq/1, Display/1, Product/2
  Gain4/1 -> Integrator1/1, Display4/1
  Add1/1 -> Gain4/1
  Vq/1 -> Add1/1
  Gain2/1 -> Add/3
  Product/1 -> Gain2/1
  wr/1 -> Display2/1, Product1/2, Gain6/1, Product/1
  Gain1/1 -> Add/2
  Integrator/1 -> Id/1, Display1/1, [Id], Gain1/1
  Gain/1 -> Display3/1, Integrator/1
  Add/1 -> Gain/1
  Vd/1 -> Add/1

== system Testing_model/Subsystem1/Park and Clark transformation1 ==
  Va : Inport
  Vb : Inport  Port=2
  Vc : Inport  Port=3
  Theta : Inport  Port=4
  Display{,1..7} (8 alike) : Display
  Subsystem : Subsystem
  Subsystem1 : Subsystem
  Vd : Outport
  Vq : Outport  Port=2
  wires:
  Theta/1 -> Subsystem1/1(Theta), Display7/1
  Subsystem1/2(Vq) -> Display1/1, Vq/1
  Subsystem1/1(Vd) -> Vd/1, Display/1
  Subsystem/2(Vbeta) -> Subsystem1/3(Vbeta), Display3/1
  Subsystem/1(Valpha) -> Subsystem1/2(Valpha), Display2/1
  Vc/1 -> Subsystem/3(In3), Display6/1
  Vb/1 -> Subsystem/2(In2), Display5/1
  Va/1 -> Subsystem/1(In1), Display4/1

== system Testing_model/Subsystem1/Speed1 ==
  Te : Inport
  TL : Inport  Port=2
  Add : Sum  Inputs=+---
  Constant : Constant  Value=2*pi
  Constant1 : Constant  Value=.03
  Display : Display
  Display1 : Display
  Gain : Gain  Gain=1/J
  Gain1 : Gain  Gain=B
  Gain2 : Gain  Gain=P
  Integrator : Integrator
  Integrator2 : Integrator
  Rem : Math  Operator=rem
  Scope : Scope
  wr : Outport
  Theta : Outport  Port=2
  wires:
  Constant1/1 -> Add/3
  Rem/1 -> Scope/1, Theta/1, Display/1
  Constant/1 -> Rem/2
  Integrator2/1 -> Rem/1
  Gain2/1 -> wr/1, Integrator2/1, Display1/1
  Gain1/1 -> Add/4
  Add/1 -> Gain/1
  TL/1 -> Add/2
  Gain/1 -> Integrator/1
  Te/1 -> Add/1
  Integrator/1 -> Gain1/1, Gain2/1

== system Testing_model/Subsystem1/Torque 1 ==
  Id : Inport
  Iq : Inport  Port=2
  Display : Display
  Display1 : Display
  Gain : Gain  Gain=lamdaM
  Gain1 : Gain  Gain=P
  Gain2 : Gain  Gain=3/2
  Gain3 : Gain
  Saturation : Saturate  UpperLimit=3.82  LowerLimit=-3.82
  Te : Outport
  wires:
  Gain3/1 -> Te/1
  Gain1/1 -> Gain2/1
  Gain2/1 -> Saturation/1
  Gain/1 -> Gain1/1
  Iq/1 -> Gain/1, Display1/1
  Saturation/1 -> Gain3/1, Display/1

== system Testing_model/Subsystem2/Forward Clacke ==
  Ia : Inport
  Ib : Inport  Port=2
  Ic : Inport  Port=3
  Gain : Gain  Gain=0.5
  Gain1 : Gain  Gain=0.5
  Gain2 : Gain  Gain=2/3
  Gain3 : Gain  Gain=sqrt(3)/2
  Gain4 : Gain  Gain=2/3
  Sum : Sum  Inputs=+--
  Sum1 : Sum  Inputs=+-
  I_alpha : Outport
  I_beta : Outport  Port=2
  wires:
  Ib/1 -> Gain/1, Sum1/1
  Gain/1 -> Sum/2
  Gain2/1 -> I_alpha/1
  Sum1/1 -> Gain3/1
  Gain1/1 -> Sum/3
  Ic/1 -> Gain1/1, Sum1/2
  Sum/1 -> Gain2/1
  Gain3/1 -> Gain4/1
  Ia/1 -> Sum/1
  Gain4/1 -> I_beta/1

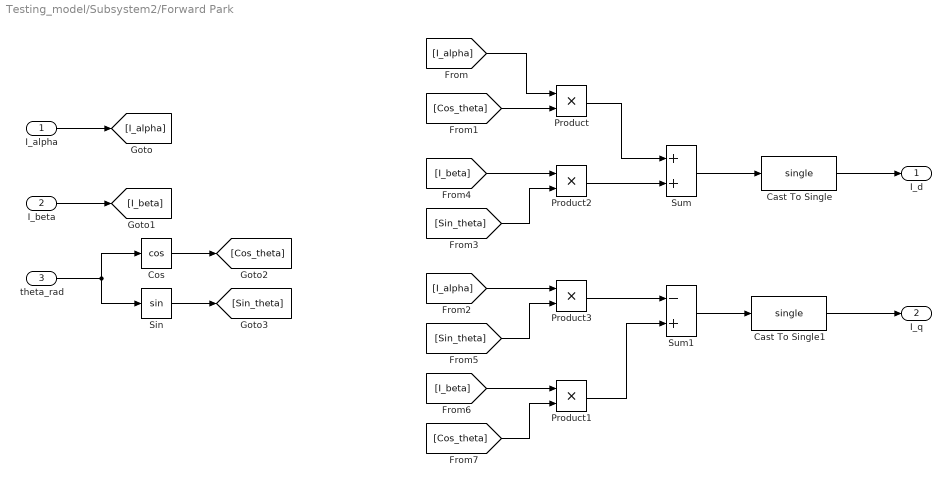
== system Testing_model/Subsystem2/Forward Park ==
  I_alpha : Inport
  I_beta : Inport  Port=2
  theta_rad : Inport  Port=3
  Cast To Single : DataTypeConversion  OutDataTypeStr=single  SaturateOnIntegerOverflow=off  RndMeth=Floor
  Cast To Single1 : DataTypeConversion  OutDataTypeStr=single  SaturateOnIntegerOverflow=off  RndMeth=Floor
  Cos : Trigonometry  Operator=cos
  Product{,1..3} (4 alike) : Product
  Sin : Trigonometry
  Sum : Sum
  Sum1 : Sum  Inputs=-+
  I_d : Outport
  I_q : Outport  Port=2
  wires:
  [Cos_theta] -> Product1/2
  [I_beta] -> Product1/1
  [Sin_theta] -> Product3/2
  [I_alpha] -> Product3/1
  Product1/1 -> Sum1/2
  [I_beta] -> Product2/1
  [Sin_theta] -> Product2/2
  [Cos_theta] -> Product/2
  Sin/1 -> [Sin_theta]
  Cos/1 -> [Cos_theta]
  theta_rad/1 -> Cos/1, Sin/1
  [I_alpha] -> Product/1
  I_beta/1 -> [I_beta]
  I_alpha/1 -> [I_alpha]
  Product3/1 -> Sum1/1
  Product2/1 -> Sum/2
  Product/1 -> Sum/1
  Sum1/1 -> Cast To Single1/1
  Sum/1 -> Cast To Single/1
  Cast To Single/1 -> I_d/1
  Cast To Single1/1 -> I_q/1

== system Testing_model/Subsystem5/Forward Clacke ==
  Ia : Inport
  Ib : Inport  Port=2
  Ic : Inport  Port=3
  Gain : Gain  Gain=0.5
  Gain1 : Gain  Gain=0.5
  Gain2 : Gain  Gain=2/3
  Gain3 : Gain  Gain=sqrt(3)/2
  Gain4 : Gain  Gain=2/3
  Sum : Sum  Inputs=+--
  Sum1 : Sum  Inputs=+-
  I_alpha : Outport
  I_beta : Outport  Port=2
  wires:
  Gain4/1 -> I_beta/1
  Ia/1 -> Sum/1
  Gain3/1 -> Gain4/1
  Sum/1 -> Gain2/1
  Ic/1 -> Sum1/2, Gain1/1
  Gain1/1 -> Sum/3
  Sum1/1 -> Gain3/1
  Gain2/1 -> I_alpha/1
  Gain/1 -> Sum/2
  Ib/1 -> Sum1/1, Gain/1

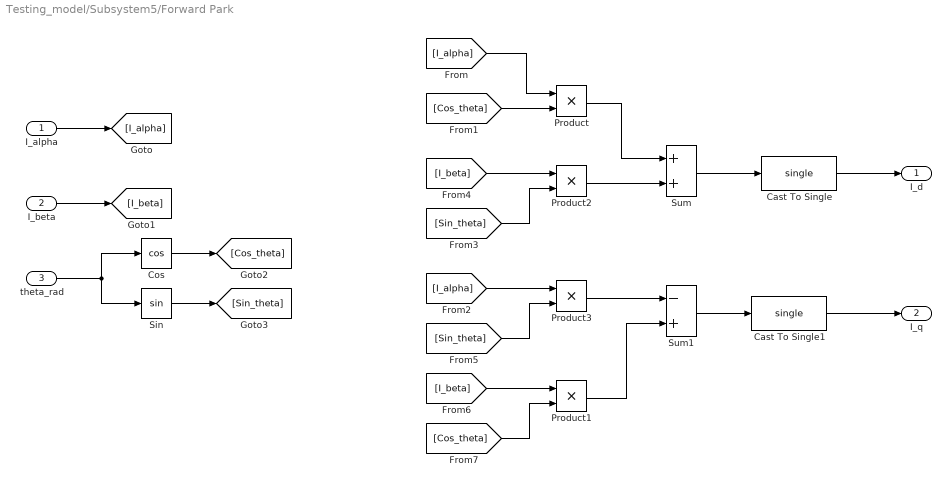
== system Testing_model/Subsystem5/Forward Park ==
  I_alpha : Inport
  I_beta : Inport  Port=2
  theta_rad : Inport  Port=3
  Cast To Single : DataTypeConversion  OutDataTypeStr=single  SaturateOnIntegerOverflow=off  RndMeth=Floor
  Cast To Single1 : DataTypeConversion  OutDataTypeStr=single  SaturateOnIntegerOverflow=off  RndMeth=Floor
  Cos : Trigonometry  Operator=cos
  Product{,1..3} (4 alike) : Product
  Sin : Trigonometry
  Sum : Sum
  Sum1 : Sum  Inputs=-+
  I_d : Outport
  I_q : Outport  Port=2
  wires:
  Cast To Single1/1 -> I_q/1
  Cast To Single/1 -> I_d/1
  Sum/1 -> Cast To Single/1
  Sum1/1 -> Cast To Single1/1
  Product/1 -> Sum/1
  Product2/1 -> Sum/2
  Product3/1 -> Sum1/1
  I_alpha/1 -> [I_alpha]
  I_beta/1 -> [I_beta]
  [I_alpha] -> Product/1
  theta_rad/1 -> Sin/1, Cos/1
  Cos/1 -> [Cos_theta]
  Sin/1 -> [Sin_theta]
  [Cos_theta] -> Product/2
  [Sin_theta] -> Product2/2
  [I_beta] -> Product2/1
  Product1/1 -> Sum1/2
  [I_alpha] -> Product3/1
  [Sin_theta] -> Product3/2
  [I_beta] -> Product1/1
  [Cos_theta] -> Product1/2

== system Testing_model/Subsystem/Inverse Transformation/Inverse Park  ==
  In1 : Inport
  In2 : Inport  Port=2
  In3 : Inport  Port=3
  Cos : Trigonometry  Operator=cos
  Cos1 : Trigonometry  Operator=cos
  Product{,1..3} (4 alike) : Product
  Sin : Trigonometry
  Sin1 : Trigonometry
  Subtract : Sum  Inputs=+-
  Subtract2 : Sum
  Valpha : Outport
  Vbeta : Outport  Port=2
  wires:
  Product3/1 -> Subtract2/1
  In3/1 -> Product2/2, Product1/2
  In1/1 -> Cos/1, [theta], Sin/1
  Subtract/1 -> Valpha/1  "Valpha"
  Product/1 -> Subtract/1
  Subtract2/1 -> Vbeta/1  "Vbeta"
  Product2/1 -> Subtract2/2
  Cos/1 -> Product/1
  Product1/1 -> Subtract/2
  [theta] -> Cos1/1
  In2/1 -> Product/2, Product3/1
  [theta] -> Sin1/1
  Sin/1 -> Product1/1
  Cos1/1 -> Product2/1
  Sin1/1 -> Product3/2

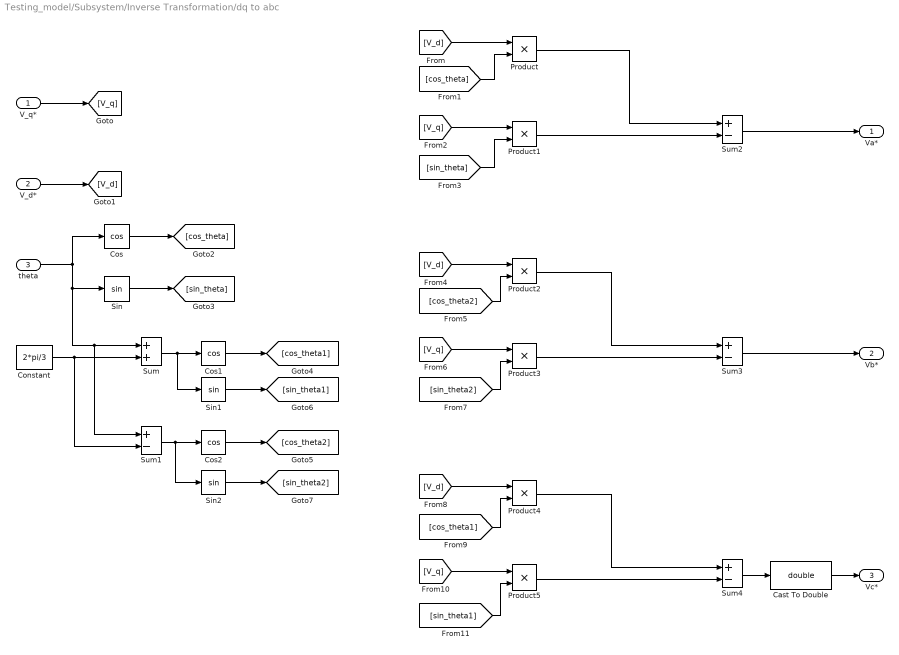
== system Testing_model/Subsystem/Inverse Transformation/dq to abc ==
  V_q* : Inport
  V_d* : Inport  Port=2
  theta : Inport  Port=3
  Cast To Double : DataTypeConversion  OutDataTypeStr=double  SaturateOnIntegerOverflow=off  RndMeth=Floor
  Constant : Constant  Value=2*pi/3
  Cos : Trigonometry  Operator=cos
  Cos1 : Trigonometry  Operator=cos
  Cos2 : Trigonometry  Operator=cos
  Product{,1..5} (6 alike) : Product
  Sin : Trigonometry
  Sin1 : Trigonometry
  Sin2 : Trigonometry
  Sum : Sum
  Sum{1..4} (4 alike) : Sum  Inputs=+-
  Va* : Outport
  Vb* : Outport  Port=2
  Vc* : Outport  Port=3
  wires:
  [sin_theta1] -> Product5/2
  [V_q] -> Product5/1
  [cos_theta1] -> Product4/2
  [V_d] -> Product4/1
  Product4/1 -> Sum4/1
  Product5/1 -> Sum4/2
  Sum4/1 -> Cast To Double/1
  [sin_theta2] -> Product3/2
  Sin2/1 -> [sin_theta2]
  Sin1/1 -> [sin_theta1]
  [V_q] -> Product3/1
  [cos_theta2] -> Product2/2
  [V_d] -> Product2/1
  Sum3/1 -> Vb*/1
  Product3/1 -> Sum3/2
  Product2/1 -> Sum3/1
  [sin_theta] -> Product1/2
  [V_q] -> Product1/1
  [cos_theta] -> Product/2
  [V_d] -> Product/1
  Product/1 -> Sum2/1
  Product1/1 -> Sum2/2
  Sum2/1 -> Va*/1
  Cos2/1 -> [cos_theta2]
  Cos1/1 -> [cos_theta1]
  Sum1/1 -> Cos2/1, Sin2/1
  Sum/1 -> Cos1/1, Sin1/1
  Constant/1 -> Sum/2, Sum1/2
  Sin/1 -> [sin_theta]
  Cos/1 -> [cos_theta]
  theta/1 -> Cos/1, Sin/1, Sum1/1, Sum/1
  V_d*/1 -> [V_d]
  V_q*/1 -> [V_q]
  Cast To Double/1 -> Vc*/1

== system Testing_model/Subsystem/Inverse Transformation/inverse Clark ==
  In1 : Inport
  In2 : Inport  Port=2
  Add : Sum
  Add1 : Sum
  Constant : Constant  Value=-1/2
  Constant1 : Constant  Value=sqrt(3)/2
  Constant2 : Constant  Value=-1/2
  Constant3 : Constant  Value=-sqrt(3)/2
  Product{,1..3} (4 alike) : Product
  Va : Outport
  Vb : Outport  Port=2
  Vc : Outport  Port=3
  wires:
  In1/1 -> Va/1, Product1/2, Product2/2
  In2/1 -> Product/1, Product3/2
  Add/1 -> Vb/1
  Product3/1 -> Add1/2
  Constant/1 -> Product1/1
  Constant2/1 -> Product2/1
  Product/1 -> Add/2
  Constant1/1 -> Product/2
  Product1/1 -> Add/1
  Product2/1 -> Add1/1
  Add1/1 -> Vc/1
  Constant3/1 -> Product3/1

== system Testing_model/Subsystem/voltage limits by maintaining the same ration/Normal_Voltage ==
  Vq_ref_new : Inport
  Vd_ref_new : Inport  Port=2
  Action Port : ActionPort  ActionPortLabel=if(u1 <= 0)
  Data Type Conversion : DataTypeConversion  OutDataTypeStr=single  SaturateOnIntegerOverflow=off  RndMeth=Floor
  Data Type Conversion1 : DataTypeConversion  OutDataTypeStr=single  SaturateOnIntegerOverflow=off  RndMeth=Floor
  Vq_ref_1 : Outport
  Vd_ref_1 : Outport  Port=2
  wires:
  Vq_ref_new/1 -> Data Type Conversion/1
  Vd_ref_new/1 -> Data Type Conversion1/1
  Data Type Conversion/1 -> Vq_ref_1/1
  Data Type Conversion1/1 -> Vd_ref_1/1

== system Testing_model/Subsystem/voltage limits by maintaining the same ration/Voltage_to_be_Limited ==
  Vq_ref_new : Inport
  Vd_ref_new : Inport  Port=2
  Action Port : ActionPort  ActionPortLabel=else
  Divide1 : Product  Inputs=*/  OutDataTypeStr=single
  Divide2 : Product  Inputs=/*  OutDataTypeStr=single
  Gain : Gain  Gain=sqrt(3)
  Gain1 : Gain  Gain=Vdc * ma
  Gain2 : Gain  Gain=Vdc * ma
  Square : Math  Operator=square  OutDataTypeStr=single
  Square Root : Sqrt  OutDataTypeStr=single  IntermediateResultsDataTypeStr=single
  Square1 : Math  Operator=square  OutDataTypeStr=single
  Sum : Sum  OutDataTypeStr=single  AccumDataTypeStr=single
  Vq_ref_2 : Outport
  Vd_ref_2 : Outport  Port=2
  wires:
  Vq_ref_new/1 -> Gain1/1, Square/1
  Sum/1 -> Square Root/1
  Vd_ref_new/1 -> Square1/1, Gain2/1
  Square1/1 -> Sum/2
  Square/1 -> Sum/1
  Divide1/1 -> Vq_ref_2/1
  Square Root/1 -> Gain/1
  Divide2/1 -> Vd_ref_2/1
  Gain/1 -> Divide2/1, Divide1/2
  Gain1/1 -> Divide1/1
  Gain2/1 -> Divide2/2

== system Testing_model/Subsystem1/Park and Clark transformation1/Subsystem ==
  In1 : Inport
  In2 : Inport  Port=2
  In3 : Inport  Port=3
  Add : Sum  Inputs=+--
  Add1 : Sum  Inputs=+-
  Gain : Gain  Gain=2/3
  Gain1 : Gain  Gain=1/2
  Gain2 : Gain  Gain=1/2
  Gain3 : Gain  Gain=sqrt(3)/2
  Gain4 : Gain  Gain=sqrt(3)/2
  Gain5 : Gain  Gain=2/3
  Valpha : Outport
  Vbeta : Outport  Port=2
  wires:
  In1/1 -> Add/1
  Gain/1 -> Valpha/1
  Add1/1 -> Gain5/1
  Add/1 -> Gain/1
  In3/1 -> Gain4/1, Gain1/1
  Gain4/1 -> Add1/2
  Gain5/1 -> Vbeta/1
  In2/1 -> Gain3/1, Gain2/1
  Gain2/1 -> Add/2
  Gain1/1 -> Add/3
  Gain3/1 -> Add1/1

== system Testing_model/Subsystem1/Park and Clark transformation1/Subsystem1 ==
  Theta : Inport
  Valpha : Inport  Port=2
  Vbeta : Inport  Port=3
  Add : Sum
  Add1 : Sum
  Cos : Trigonometry  Operator=cos
  Cos1 : Trigonometry  Operator=cos
  Gain : Gain  Gain=-1
  Product{,1..3} (4 alike) : Product
  Sin : Trigonometry
  Sin1 : Trigonometry
  Vd : Outport
  Vq : Outport  Port=2
  wires:
  Add1/1 -> Vq/1
  Valpha/1 -> Product/2, [Valpha]
  Add/1 -> Vd/1
  [Valpha] -> Product3/1
  Vbeta/1 -> Product1/2, Product2/1
  Product2/1 -> Add1/1
  Product3/1 -> Add1/2
  Cos/1 -> Product/1
  Cos1/1 -> Product2/2
  [Theta] -> Cos1/1, Sin1/1
  Product1/1 -> Add/1
  Theta/1 -> Sin/1, Cos/1, [Theta]
  Sin/1 -> Product1/1
  Product/1 -> Add/2
  Gain/1 -> Product3/2
  Sin1/1 -> Gain/1
